simulink subsystem "LedsBitsDJ"  (R2022b)
settings: Solver=VariableStepAuto  StartTime=0.0  StopTime=10.0  RelTol=1e-3
libraries: arduinolib x3, simulink x1
settings Model: Creator=dar.io  LastModifiedBy=dar.io

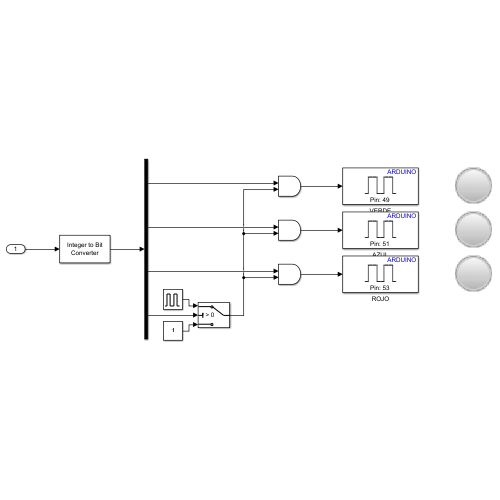
[thumbnail: Simulink's stored preview of the top-level diagram]
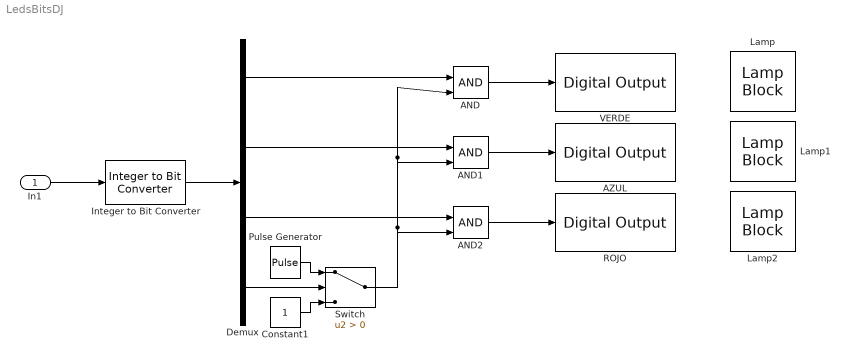
== system LedsBitsDJ ==
  In1 : Inport  OutDataTypeStr=uint8
  AND : Logic  IconShape=distinctive  AllPortsSameDT=off  OutDataTypeStr=boolean
  AND1 : Logic  IconShape=distinctive  AllPortsSameDT=off  OutDataTypeStr=boolean
  AND2 : Logic  IconShape=distinctive  AllPortsSameDT=off  OutDataTypeStr=boolean
  AZUL : arduinolib/Digital Output  pinNumber=51  Direction=output  blockPlatform=arduino
  Constant1 : Constant
  Demux : Demux
  Integer to Bit Converter : simulink/Logic and Bit Operations/Integer to Bit Converter  nbits=4  signedInputValues=Unsigned  bitOrder=LSB first  outDtype=Inherit via internal rule
  Lamp : LampBlock  LabelPosition=Hide
  Lamp1 : LampBlock  LabelPosition=Hide
  Lamp2 : LampBlock  LabelPosition=Hide
  Pulse Generator : DiscretePulseGenerator  PulseType=Time based  Period=10  PulseWidth=5
  ROJO : arduinolib/Digital Output  pinNumber=53  Direction=output  blockPlatform=arduino
  Switch : Switch  Criteria=u2 > Threshold  SaturateOnIntegerOverflow=off  InputSameDT=off
  VERDE : arduinolib/Digital Output  pinNumber=49  Direction=output  blockPlatform=arduino
  wires:
  In1/1 -> Integer to Bit Converter/1
  Demux/1 -> AND/1
  AND/1 -> VERDE/1
  Pulse Generator/1 -> Switch/1
  Integer to Bit Converter/1 -> Demux/1
  Demux/2 -> AND1/1
  Demux/3 -> AND2/1
  Constant1/1 -> Switch/3
  Switch/1 -> AND2/2, AND1/2, AND/2
  Demux/4 -> Switch/2
  AND2/1 -> ROJO/1
  AND1/1 -> AZUL/1
